simulink model "p3"  (R2020a)
settings: Solver=VariableStepAuto  StartTime=0.0  StopTime=10.0  RelTol=1e-3
undefined symbols (not defined in the file): downtab, downth, emap, Iei, Iv, Kfactor, N20, nevec, Rfd, rload0, rload2, Rw, sigbuilder_block, speedratio, thvec, Torkratio, uptab, upth
settings Model: Creator=007  LastModifiedBy=007

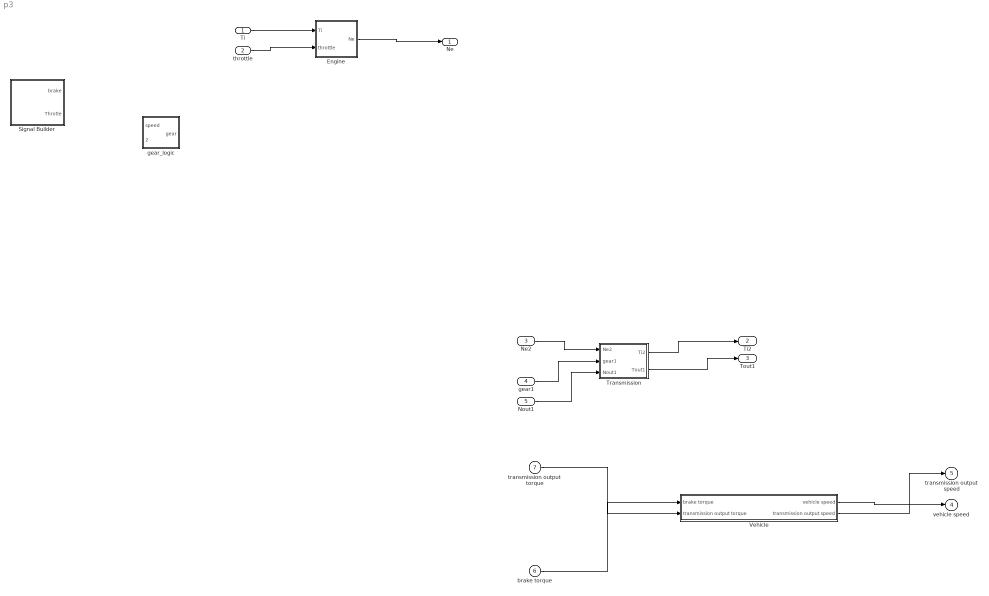
== system p3 ==
  Ti : Inport
  throttle : Inport  Port=2
  Ne2 : Inport  Port=3
  gear1 : Inport  Port=4
  Nout1 : Inport  Port=5
  brake torque : Inport  Port=6
  transmission output torque : Inport  Port=7
  Engine : Subsystem
  Signal Builder : Subsystem  Tag=STV Subsys  LoadFcn=sigbuilder_block('load');  StartFcn=sigbuilder_block('start');  StopFcn=sigbuilder_block('stop');  ClipboardFcn=sigbuilder_block('clipboard');  mask(Sigbuilder block){tuvar=[0:10]}
      mask help: Simulink:masks:SigbuilderBlock_MD
      mask init:
      | if ~strcmp(get_param(bdroot(gcbh),'SimulationStatus'),'stopped') tuvar = sigbuilder_block('maskInit'); end
      settings: CopyFcn=sigbuilder_block('copy');  DeleteFcn=sigbuilder_block('delete');  ModelCloseFcn=sigbuilder_block('modelClose');  PreSaveFcn=sigbuilder_block('preSave');  PauseFcn=sigbuilder_block('pause');  ContinueFcn=sigbuilder_block('continue');  NameChangeFcn=sigbuilder_block('namechange');  OpenFcn=sigbuilder_block('open',[437.6 153 550.4 359.25 ]);  CloseFcn=sigbuilder_block('close');
      mask Display: plot(0, 0, 100, 100,[2, 2, 32, 32, 2], [68, 8, 8, 68, 68],[32, 2], [38, 38], [32, 19, 2],[53, 60, 44], [32, 17, 17, 2],[16, 16, 31, 31]);txt = getActiveGroup(gcbh);text(2, 100, txt,'verticalAlignment', 'top');
  Transmission : Subsystem
  Vehicle : Subsystem
  gear_logic : Stateflow chart  TreatAsAtomicUnit=on
  Ne : Outport  VectorParamsAs1DForOutWhenUnconnected=off
  Ti2 : Outport  Port=2  VectorParamsAs1DForOutWhenUnconnected=off
  Tout1 : Outport  Port=3  VectorParamsAs1DForOutWhenUnconnected=off
  vehicle speed : Outport  Port=4  VectorParamsAs1DForOutWhenUnconnected=off
  transmission output speed : Outport  Port=5  VectorParamsAs1DForOutWhenUnconnected=off
  wires:
  Ti/1 -> Engine/1(Ti)
  throttle/1 -> Engine/2(throttle)
  Engine/1(Ne) -> Ne/1
  Ne2/1 -> Transmission/1(Ne2)
  gear1/1 -> Transmission/2(gear1)
  Nout1/1 -> Transmission/3(Nout1)
  Transmission/1(Ti2) -> Ti2/1
  Transmission/2(Tout1) -> Tout1/1
  brake torque/1 -> Vehicle/1(brake torque)
  transmission output torque/1 -> Vehicle/2(transmission output torque)
  Vehicle/1(vehicle speed) -> vehicle speed/1
  Vehicle/2(transmission output speed) -> transmission output speed/1

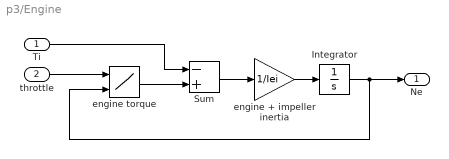
== system p3/Engine ==
  Ti : Inport
  throttle : Inport  Port=2
  Integrator : Integrator  InitialCondition=1000  LimitOutput=on  UpperSaturationLimit=6000  LowerSaturationLimit=600  ZeroCross=off
  Sum : Sum  Inputs=-+  InputSameDT=on  SaturateOnIntegerOverflow=on  OutDataTypeStr=Inherit: Same as first input
  engine torque : Lookup_n-D  BreakpointsForDimension1=thvec  BreakpointsForDimension2=nevec  Table=emap  InternalRulePriority=Speed  InputSameDT=on
  engine + impeller inertia : Gain  Gain=1/Iei  SaturateOnIntegerOverflow=on  OutDataTypeStr=Inherit: Same as input  ParamDataTypeStr=Inherit: Same as input
  Ne : Outport  VectorParamsAs1DForOutWhenUnconnected=off
  wires:
  throttle/1 -> engine torque/1
  Ti/1 -> Sum/1
  engine + impeller inertia/1 -> Integrator/1
  Integrator/1 -> Ne/1, engine torque/2
  engine torque/1 -> Sum/2
  Sum/1 -> engine + impeller inertia/1

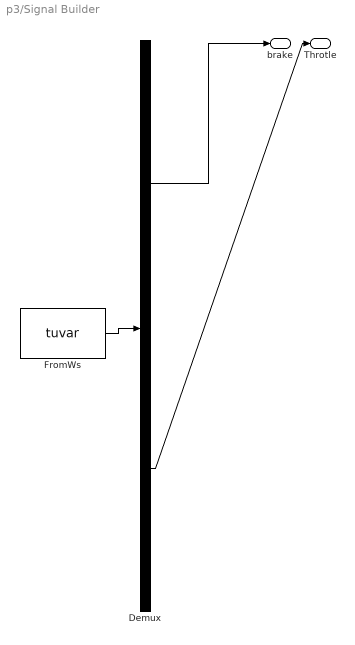
== system p3/Signal Builder ==
  Demux : Demux  Tag=STV Demux  Outputs=2
      settings: DisplayOption=none
  FromWs : FromWorkspace  Tag=STV FromWs  VariableName=tuvar
      SigBuilderData=|
      | common.afterFinalStr = 'Extrapolate'
      | common.sampleTime = 0
      | dataSet.timeRange = [0 10]
      | dataSet.name = 'Group 1'
      | sbobj.Groups.Name = 'Group 1'
      | sbobj.Groups.Signals(1).Name = 'brake'
      | sbobj.Groups.Signals(1).XData = [0 4 4 6 6 10]
      | sbobj.Groups.Signals(1).YData = [0 0 1 1 0 0]
      | sbobj.Groups.Signals(2).Name = 'Throtle'
      | sbobj.Groups.Signals(2).XData = [0 10]
      | sbobj.Groups.Signals(2).YData = [0 0]
  brake : Outport  Tag=STV Outport
  Throtle : Outport  Tag=STV Outport  Port=2
  wires:
  Demux/1 -> brake/1
  FromWs/1 -> Demux/1
  Demux/2 -> Throtle/1

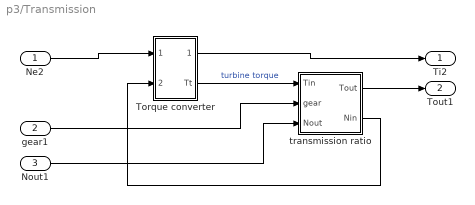
== system p3/Transmission ==
  Ne2 : Inport
  gear1 : Inport  Port=2
  Nout1 : Inport  Port=3
  Torque converter : Subsystem
  transmission ratio : Subsystem
  Ti2 : Outport  VectorParamsAs1DForOutWhenUnconnected=off
  Tout1 : Outport  Port=2  VectorParamsAs1DForOutWhenUnconnected=off
  wires:
  transmission ratio/2(Nin) -> Torque converter/2(Nin1)
  Torque converter/2(Tt) -> transmission ratio/1(Tin)  "turbine torque"
  gear1/1 -> transmission ratio/2(gear)
  Nout1/1 -> transmission ratio/3(Nout)
  Torque converter/1(Ti1) -> Ti2/1
  transmission ratio/1(Tout) -> Tout1/1
  Ne2/1 -> Torque converter/1(Ne1)

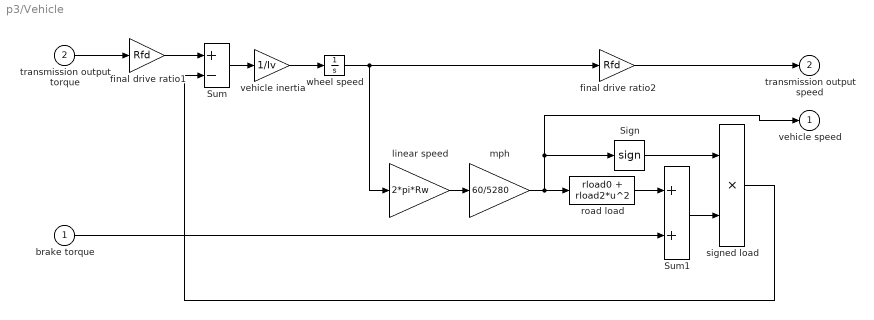
== system p3/Vehicle ==
  brake torque : Inport
  transmission output torque : Inport  Port=2
  Sign : Signum
  Sum : Sum  Inputs=+-  InputSameDT=on  SaturateOnIntegerOverflow=on  OutDataTypeStr=Inherit: Same as first input
  Sum1 : Sum  InputSameDT=on  SaturateOnIntegerOverflow=on  OutDataTypeStr=Inherit: Same as first input
  final drive ratio1 : Gain  Gain=Rfd  SaturateOnIntegerOverflow=on  OutDataTypeStr=Inherit: Same as input  ParamDataTypeStr=Inherit: Same as input
  final drive ratio2 : Gain  Gain=Rfd  SaturateOnIntegerOverflow=on  OutDataTypeStr=Inherit: Same as input  ParamDataTypeStr=Inherit: Same as input
  linear speed : Gain  Gain=2*pi*Rw  SaturateOnIntegerOverflow=on  OutDataTypeStr=Inherit: Same as input  ParamDataTypeStr=Inherit: Same as input
  mph : Gain  Gain=60/5280  SaturateOnIntegerOverflow=on  OutDataTypeStr=Inherit: Same as input  ParamDataTypeStr=Inherit: Same as input
  road load : Fcn  Expr=rload0 + rload2*u^2
  signed load : Product  InputSameDT=on  SaturateOnIntegerOverflow=on  OutDataTypeStr=Inherit: Same as first input
  vehicle inertia : Gain  Gain=1/Iv  SaturateOnIntegerOverflow=on  OutDataTypeStr=Inherit: Same as input  ParamDataTypeStr=Inherit: Same as input
  wheel speed : Integrator  InitialCondition=N20/Rfd  ZeroCross=off
  vehicle speed : Outport  VectorParamsAs1DForOutWhenUnconnected=off
  transmission output speed : Outport  Port=2  VectorParamsAs1DForOutWhenUnconnected=off
  wires:
  vehicle inertia/1 -> wheel speed/1
  road load/1 -> Sum1/1
  linear speed/1 -> mph/1
  mph/1 -> vehicle speed/1, Sign/1, road load/1
  final drive ratio1/1 -> Sum/1
  wheel speed/1 -> linear speed/1, final drive ratio2/1
  Sign/1 -> signed load/1
  Sum/1 -> vehicle inertia/1
  signed load/1 -> Sum/2
  final drive ratio2/1 -> transmission output speed/1
  transmission output torque/1 -> final drive ratio1/1
  Sum1/1 -> signed load/2
  brake torque/1 -> Sum1/2

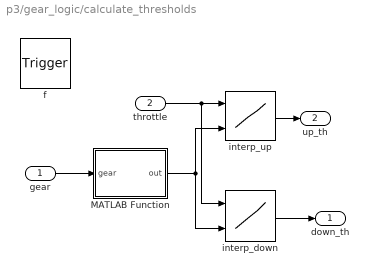
== system p3/gear_logic/calculate_thresholds ==
  gear : Inport  OutDataTypeStr=double  PortDimensions=1
  throttle : Inport  Port=2  OutDataTypeStr=double  PortDimensions=1
  f : TriggerPort  TriggerType=function-call  VariantControl=(inherit)
      settings: CopyFcn=Stateflow.SLINSF.SimulinkMan.removeBlockPreDeleteFcn  PreDeleteFcn=Stateflow.SLINSF.SimulinkMan.unsafePredeleteFcn
  MATLAB Function : MATLAB Function  TreatAsAtomicUnit=on
  interp_down : Lookup_n-D  BreakpointsForDimension1=downth  BreakpointsForDimension2=[1:4]  Table=downtab  InputSameDT=on
  interp_up : Lookup_n-D  BreakpointsForDimension1=upth  BreakpointsForDimension2=[1:4]  Table=uptab  InputSameDT=on
  down_th : Outport
  up_th : Outport  Port=2
  wires:
  gear/1 -> MATLAB Function/1(gear)
  MATLAB Function/1(out) -> interp_up/2, interp_down/2
  throttle/1 -> interp_down/1, interp_up/1
  interp_up/1 -> up_th/1
  interp_down/1 -> down_th/1

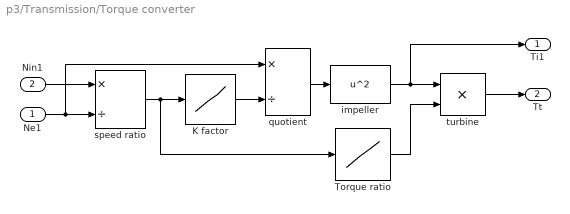
== system p3/Transmission/Torque converter ==
  Ne1 : Inport
  Nin1 : Inport  Port=2
  K factor : Lookup_n-D  NumberOfTableDimensions=1  BreakpointsForDimension1=speedratio  Table=Kfactor  InternalRulePriority=Speed  SaturateOnIntegerOverflow=on  InputSameDT=on
  Torque ratio : Lookup_n-D  NumberOfTableDimensions=1  BreakpointsForDimension1=speedratio  Table=Torkratio  InternalRulePriority=Speed  SaturateOnIntegerOverflow=on  InputSameDT=on
  impeller : Fcn  Expr=u^2
  quotient : Product  Inputs=*/  InputSameDT=on  SaturateOnIntegerOverflow=on  OutDataTypeStr=Inherit: Same as first input
  speed ratio : Product  Inputs=*/  InputSameDT=on  SaturateOnIntegerOverflow=on  OutDataTypeStr=Inherit: Same as first input
  turbine : Product  InputSameDT=on  SaturateOnIntegerOverflow=on  OutDataTypeStr=Inherit: Same as first input
  Ti1 : Outport  VectorParamsAs1DForOutWhenUnconnected=off
  Tt : Outport  Port=2  VectorParamsAs1DForOutWhenUnconnected=off
  wires:
  speed ratio/1 -> Torque ratio/1, K factor/1
  Ne1/1 -> speed ratio/2, quotient/1
  impeller/1 -> Ti1/1, turbine/1
  quotient/1 -> impeller/1
  Torque ratio/1 -> turbine/2
  K factor/1 -> quotient/2
  Nin1/1 -> speed ratio/1
  turbine/1 -> Tt/1

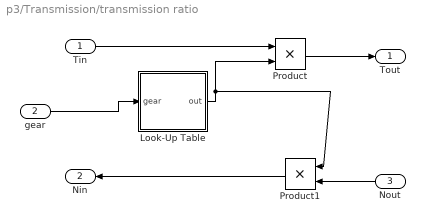
== system p3/Transmission/transmission ratio ==
  Tin : Inport
  gear : Inport  Port=2
  Nout : Inport  Port=3
  Look-Up Table : MATLAB Function  TreatAsAtomicUnit=on
  Product : Product  InputSameDT=on  SaturateOnIntegerOverflow=on  OutDataTypeStr=Inherit: Same as first input
  Product1 : Product  InputSameDT=on  SaturateOnIntegerOverflow=on  OutDataTypeStr=Inherit: Same as first input
  Tout : Outport  VectorParamsAs1DForOutWhenUnconnected=off
  Nin : Outport  Port=2  VectorParamsAs1DForOutWhenUnconnected=off
  wires:
  Look-Up Table/1(out) -> Product1/1, Product/2
  Nout/1 -> Product1/2
  Product1/1 -> Nin/1
  Product/1 -> Tout/1
  Tin/1 -> Product/1
  gear/1 -> Look-Up Table/1(gear)

== matlab function p3/gear_logic/calculate_thresholds/MATLAB Function ==
  data: gear input; out output
function out = fcn(gear)
    %#codegen
    table = [1 2 3 4];
    switch(gear)
        case gearType.fourth;
            out=table(4);        
        case gearType.third;
            out=table(3);
        case gearType.second;
            out=table(2);            
        otherwise; % gearType.first
            out=table(1);
    end
    
end

== stateflow chart p3/gear_logic ==
  state gear
    gear
    en,du:
    [down_threshold,up_threshold] = calculate_thresholds(gear,throttle);
    up = duration(speed >= up_threshold) > TWAIT;
    down = duration(speed <= down_threshold) > TWAIT;
    state first
    state second
    state third
    state fourth
    second -> third [order 1] : [up]
    third -> fourth [order 1] : [up]
    first -> second : [up]
    (default) -> first
    second -> first [order 2] : [down]
    third -> second [order 2] : [down]
    fourth -> third : [down]
  state [down_th,up_th] = calculate_thresholds(gear,throttle) [function]
  (default) -> gear
  data: gear function_input double size=1; throttle function_input double size=1; down_th function_output; up_th function_output; gear output; TWAIT parameter; up local; down local; speed input; throttle input; down_threshold local; up_threshold local

== matlab function p3/Transmission/transmission ratio/Look-Up Table ==
  data: gear input; out output
function out = fcn(gear)
    %#codegen
    table = [2.393 1.450 1.000 0.677];
    switch(gear)
        case gearType.fourth;
            out=table(4);        
        case gearType.third;
            out=table(3);            
        case gearType.second;
            out=table(2);
        otherwise; % gearType.first
            out=table(1);
    end
    
end
